simulink model "aula05"  (R2022a)
settings: Solver=VariableStepAuto  StartTime=0.0  StopTime=200  RelTol=1e-3
settings Model: Creator=a2150336  LastModifiedBy=a2150336

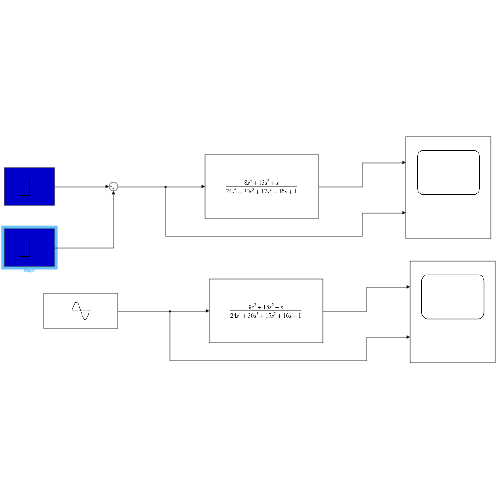
[thumbnail: Simulink's stored preview of the top-level diagram]
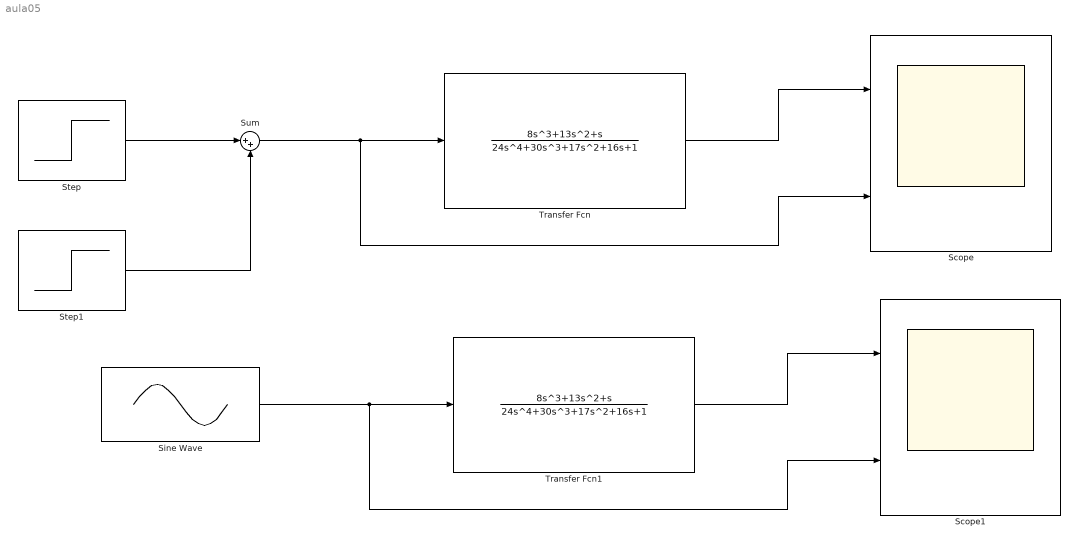
== system aula05 ==
  Scope : Scope  NumInputPorts=2
  Scope1 : Scope  NumInputPorts=2
  Sine Wave : Sin  SampleTime=0
  Step : Step  SampleTime=0
  Step1 : Step  SampleTime=0
  Sum : Sum  Inputs=|++
  Transfer Fcn : TransferFcn  Numerator=[8 13 1 0]  Denominator=[24 30 17 16 1]
  Transfer Fcn1 : TransferFcn  Numerator=[8 13 1 0]  Denominator=[24 30 17 16 1]
  wires:
  Transfer Fcn/1 -> Scope/1
  Step/1 -> Sum/1
  Sum/1 -> Scope/2, Transfer Fcn/1
  Step1/1 -> Sum/2
  Sine Wave/1 -> Scope1/2, Transfer Fcn1/1
  Transfer Fcn1/1 -> Scope1/1
